simulink subsystem "autopilot_subsystem"  (R2021b)
settings: Solver=VariableStepAuto  StartTime=0.0  StopTime=10.0  RelTol=1e-3
values from neighbouring files (symbols this model uses):
  Ka = 4.5    [PN_Guidance_matlab.m]
  Kdc = 1.12    [PN_Guidance_matlab.m]
  Ki = 14.3    [PN_Guidance_matlab.m]
  Kr = -0.37    [PN_Guidance_matlab.m]
  l_M0 = 80*d2r    (= 1.3962634016)    [PN_Guidance_matlab.m]
settings Model: Creator=rocke  LastModifiedBy=rocke

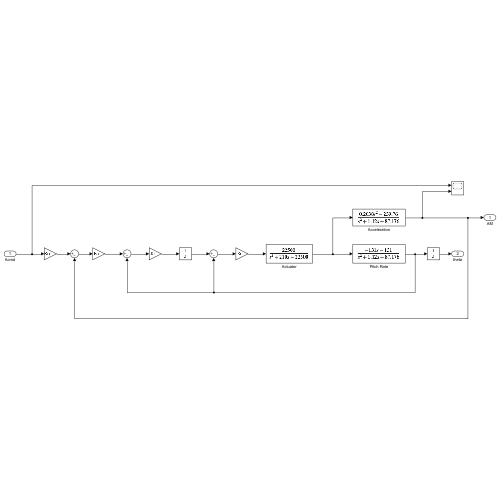
[thumbnail: Simulink's stored preview of the top-level diagram]
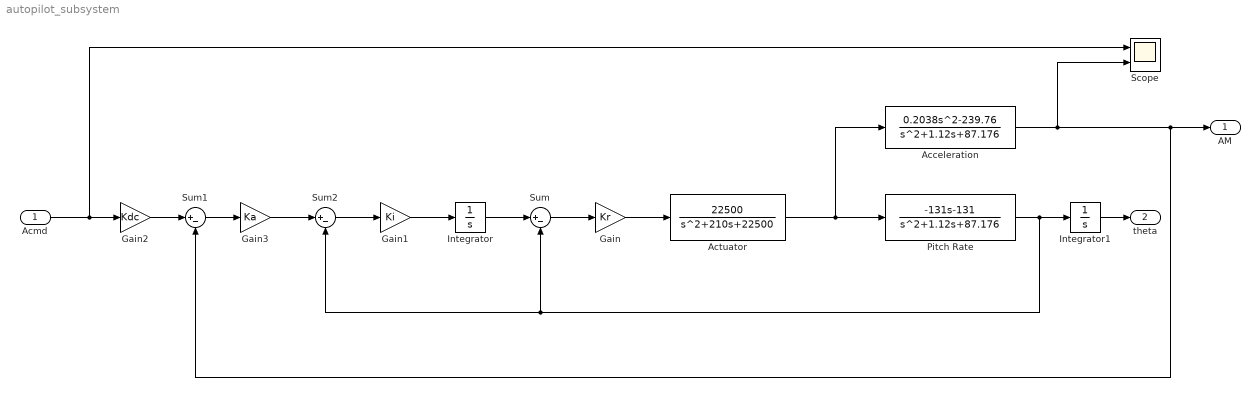
== system autopilot_subsystem ==
  Acmd : Inport
  Acceleration : TransferFcn  Numerator=[0.2038 0 -239.76]  Denominator=[1 1.12 87.176]
  Actuator : TransferFcn  Numerator=[22500]  Denominator=[1 210 22500]
  Gain : Gain  Gain=Kr
  Gain1 : Gain  Gain=Ki
  Gain2 : Gain  Gain=Kdc
  Gain3 : Gain  Gain=Ka
  Integrator : Integrator
  Integrator1 : Integrator  InitialCondition=l_M0
  Pitch Rate : TransferFcn  Numerator=[-131 -131]  Denominator=[1 1.12 87.176]
  Scope : Scope  NumInputPorts=2
  Sum : Sum  Inputs=|+-
  Sum1 : Sum  Inputs=|+-
  Sum2 : Sum  Inputs=|+-
  AM : Outport
  theta : Outport  Port=2
  wires:
  Sum1/1 -> Gain3/1
  Gain/1 -> Actuator/1
  Actuator/1 -> Acceleration/1, Pitch Rate/1
  Sum/1 -> Gain/1
  Acceleration/1 -> Scope/2, Sum1/2, AM/1
  Pitch Rate/1 -> Integrator1/1, Sum/2, Sum2/2
  Gain3/1 -> Sum2/1
  Gain1/1 -> Integrator/1
  Integrator/1 -> Sum/1
  Integrator1/1 -> theta/1
  Gain2/1 -> Sum1/1
  Acmd/1 -> Scope/1, Gain2/1
  Sum2/1 -> Gain1/1
